simulink model "PI"  (R2020a)
settings: Solver=VariableStepAuto  StartTime=0.0  StopTime=30  RelTol=1e-3
settings Model: Creator=Navid  LastModifiedBy=Navid

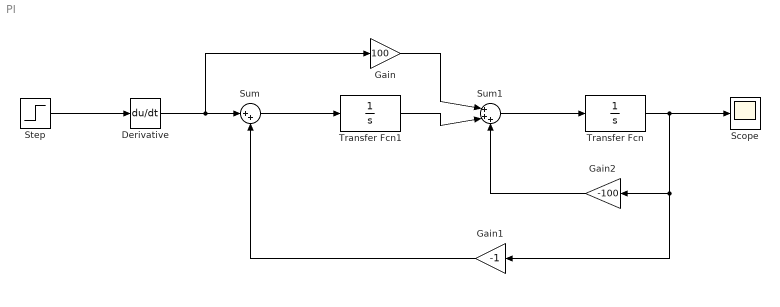
== system PI ==
  Derivative : Derivative
  Gain : Gain  Gain=100
  Gain1 : Gain  Gain=-1
  Gain2 : Gain  Gain=-100
  Scope : Scope
  Step : Step  Time=0.001  SampleTime=0
  Sum : Sum  Inputs=|++
  Sum1 : Sum  Inputs=|+++
  Transfer Fcn : TransferFcn  Denominator=[1 0]
  Transfer Fcn1 : TransferFcn  Denominator=[1 0]
  wires:
  Sum/1 -> Transfer Fcn1/1
  Sum1/1 -> Transfer Fcn/1
  Transfer Fcn/1 -> Scope/1, Gain1/1, Gain2/1
  Gain1/1 -> Sum/2
  Gain2/1 -> Sum1/3
  Transfer Fcn1/1 -> Sum1/2
  Gain/1 -> Sum1/1
  Step/1 -> Derivative/1
  Derivative/1 -> Gain/1, Sum/1
